simulink model "laby2"  (R2016a)
settings: Solver=ode23  StartTime=0.0  StopTime=10.0  RelTol=1e-5
libraries: simulink x2
settings Model: Creator=wojta  LastModifiedBy=wojta

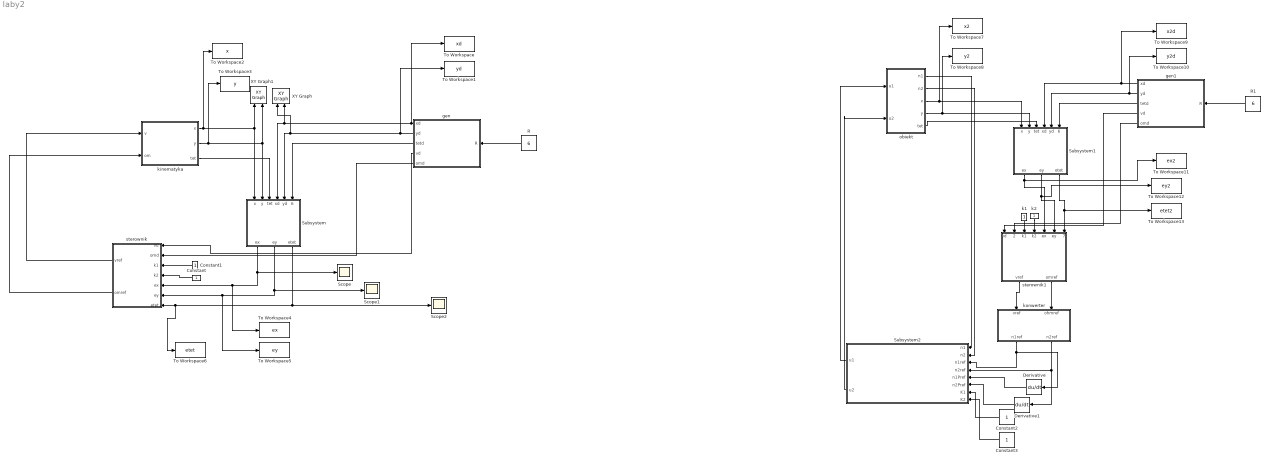
== system laby2 ==
  Constant{,1..3} (4 alike) : Constant
  Derivative : Derivative
  Derivative1 : Derivative
  R : Constant  Value=6
  R1 : Constant  Value=6
  Scope : Scope
  Scope1 : Scope
  Scope2 : Scope
  Subsystem : Subsystem
  Subsystem1 : Subsystem
  Subsystem2 : Subsystem
  To Workspace : ToWorkspace  VariableName=xd  SampleTime=-1
  To Workspace1 : ToWorkspace  VariableName=yd  SampleTime=-1
  To Workspace10 : ToWorkspace  VariableName=y2d  SampleTime=-1
  To Workspace11 : ToWorkspace  VariableName=ex2  SampleTime=-1
  To Workspace12 : ToWorkspace  VariableName=ey2  SampleTime=-1
  To Workspace13 : ToWorkspace  VariableName=etet2  SampleTime=-1
  To Workspace2 : ToWorkspace  VariableName=x  SampleTime=-1
  To Workspace3 : ToWorkspace  VariableName=y  SampleTime=-1
  To Workspace4 : ToWorkspace  VariableName=ex  SampleTime=-1
  To Workspace5 : ToWorkspace  VariableName=ey  SampleTime=-1
  To Workspace6 : ToWorkspace  VariableName=etet  SampleTime=-1
  To Workspace7 : ToWorkspace  VariableName=x2  SampleTime=-1
  To Workspace8 : ToWorkspace  VariableName=y2  SampleTime=-1
  To Workspace9 : ToWorkspace  VariableName=x2d  SampleTime=-1
  XY Graph : simulink/Sinks/XY Graph  xmin=-6  xmax=6  ymin=-6  ymax=6  st=-1
  XY Graph1 : simulink/Sinks/XY Graph  xmin=-6  xmax=6  ymin=-6  ymax=6  st=-1
  gen : Subsystem
  gen1 : Subsystem
  k1 : Constant
  k2 : Constant
  kinematyka : Subsystem
  konwerter : Subsystem
  obiekt : Subsystem
  sterownik : Subsystem
  sterownik1 : Subsystem
  wires:
  R/1 -> gen/1(R)
  sterownik/1(vref) -> kinematyka/1(v)
  sterownik/2(omref) -> kinematyka/2(om)
  kinematyka/1(x) -> To Workspace2/1, XY Graph1/1, Subsystem/1(x)
  kinematyka/2(y) -> To Workspace3/1, XY Graph1/2, Subsystem/2(y)
  kinematyka/3(tet) -> Subsystem/3(tet)
  gen/1(xd) -> To Workspace/1, XY Graph/2, Subsystem/4(xd)
  gen/2(yd) -> To Workspace1/1, XY Graph/1, Subsystem/5(yd)
  gen/3(tetd) -> Subsystem/6(tetd)
  Subsystem/1(ex) -> To Workspace4/1, sterownik/5(ex), Scope/1
  Subsystem/2(ey) -> To Workspace5/1, sterownik/6(ey), Scope1/1
  Subsystem/3(etet) -> Scope2/1, To Workspace6/1, sterownik/7(etet)
  gen/4(vd) -> sterownik/1(vd)
  gen/5(omd) -> sterownik/2(omd)
  Constant1/1 -> sterownik/3(k1)
  Constant/1 -> sterownik/4(k2)
  R1/1 -> gen1/1(R)
  k2/1 -> sterownik1/4(k2)
  k1/1 -> sterownik1/3(k1)
  Subsystem1/3(etet) -> sterownik1/7(etet), To Workspace13/1
  Subsystem1/2(ey) -> To Workspace12/1, sterownik1/6(ey)
  Subsystem1/1(ex) -> To Workspace11/1, sterownik1/5(ex)
  gen1/4(vd) -> sterownik1/1(vd)
  gen1/5(omd) -> sterownik1/2(omd)
  gen1/2(yd) -> To Workspace10/1, Subsystem1/5(yd)
  gen1/3(tetd) -> Subsystem1/6(tetd)
  obiekt/3(x) -> To Workspace7/1, Subsystem1/1(x)
  obiekt/4(y) -> To Workspace8/1, Subsystem1/2(y)
  obiekt/5(tet) -> Subsystem1/3(tet)
  sterownik1/1(vref) -> konwerter/1(vref)
  sterownik1/2(omref) -> konwerter/2(ohmref)
  konwerter/1(n1ref) -> Derivative/1, Subsystem2/3(n1ref)
  konwerter/2(n2ref) -> Derivative1/1, Subsystem2/4(n2ref)
  Derivative/1 -> Subsystem2/5(n1Pref)
  Derivative1/1 -> Subsystem2/6(n2Pref)
  Subsystem2/1(u1) -> obiekt/1(u1)
  Subsystem2/2(u2) -> obiekt/2(u2)
  obiekt/2(n2) -> Subsystem2/2(n2)
  obiekt/1(n1) -> Subsystem2/1(n1)
  Constant2/1 -> Subsystem2/7(K1)
  Constant3/1 -> Subsystem2/8(K2)
  gen1/1(xd) -> To Workspace9/1, Subsystem1/4(xd)

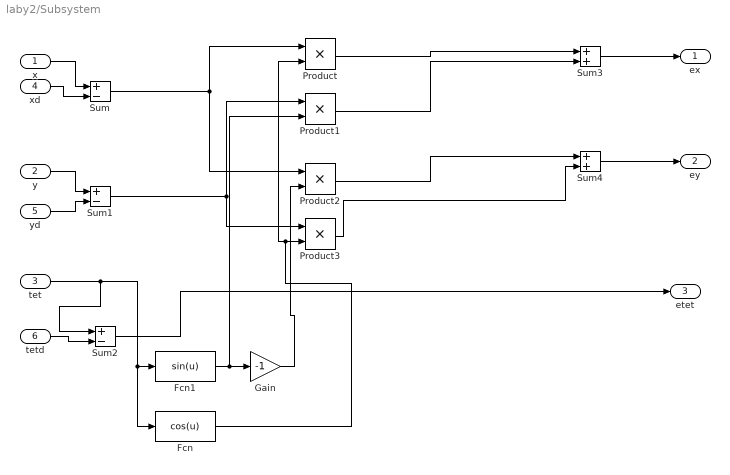
== system laby2/Subsystem ==
  x : Inport
  y : Inport  Port=2
  tet : Inport  Port=3
  xd : Inport  Port=4
  yd : Inport  Port=5
  tetd : Inport  Port=6
  Fcn : Fcn  Expr=cos(u)
  Fcn1 : Fcn  Expr=sin(u)
  Gain : Gain  Gain=-1
  Product{,1..3} (4 alike) : Product
  Sum : Sum  Inputs=+-
  Sum1 : Sum  Inputs=+-
  Sum2 : Sum  Inputs=+-
  Sum3 : Sum
  Sum4 : Sum
  ex : Outport
  ey : Outport  Port=2
  etet : Outport  Port=3
  wires:
  xd/1 -> Sum/2
  yd/1 -> Sum1/2
  Product3/1 -> Sum4/2
  tetd/1 -> Sum2/2
  Fcn1/1 -> Product1/2, Gain/1
  Product1/1 -> Sum3/2
  tet/1 -> Fcn/1, Fcn1/1, Sum2/1
  Gain/1 -> Product2/2
  Product2/1 -> Sum4/1
  Sum2/1 -> etet/1
  y/1 -> Sum1/1
  Product/1 -> Sum3/1
  Sum1/1 -> Product3/1, Product1/1
  Sum4/1 -> ey/1
  x/1 -> Sum/1
  Fcn/1 -> Product/2, Product3/2
  Sum3/1 -> ex/1
  Sum/1 -> Product/1, Product2/1

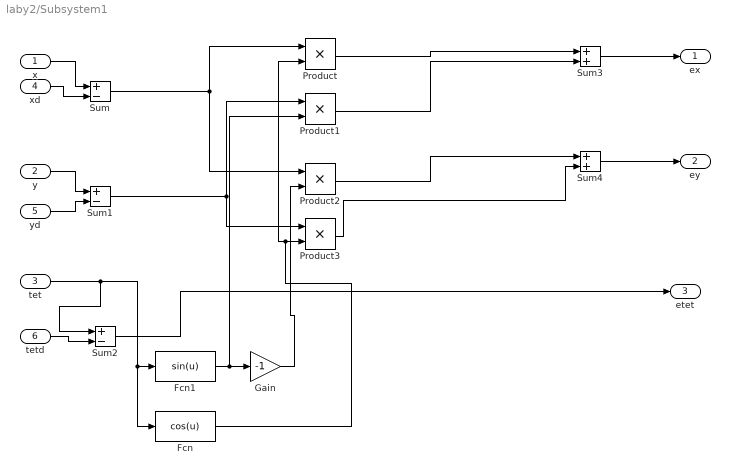
== system laby2/Subsystem1 ==
  x : Inport
  y : Inport  Port=2
  tet : Inport  Port=3
  xd : Inport  Port=4
  yd : Inport  Port=5
  tetd : Inport  Port=6
  Fcn : Fcn  Expr=cos(u)
  Fcn1 : Fcn  Expr=sin(u)
  Gain : Gain  Gain=-1
  Product{,1..3} (4 alike) : Product
  Sum : Sum  Inputs=+-
  Sum1 : Sum  Inputs=+-
  Sum2 : Sum  Inputs=+-
  Sum3 : Sum
  Sum4 : Sum
  ex : Outport
  ey : Outport  Port=2
  etet : Outport  Port=3
  wires:
  xd/1 -> Sum/2
  yd/1 -> Sum1/2
  Product3/1 -> Sum4/2
  tetd/1 -> Sum2/2
  Fcn1/1 -> Product1/2, Gain/1
  Product1/1 -> Sum3/2
  tet/1 -> Fcn/1, Fcn1/1, Sum2/1
  Gain/1 -> Product2/2
  Product2/1 -> Sum4/1
  Sum2/1 -> etet/1
  y/1 -> Sum1/1
  Product/1 -> Sum3/1
  Sum1/1 -> Product3/1, Product1/1
  Sum4/1 -> ey/1
  x/1 -> Sum/1
  Fcn/1 -> Product/2, Product3/2
  Sum3/1 -> ex/1
  Sum/1 -> Product/1, Product2/1

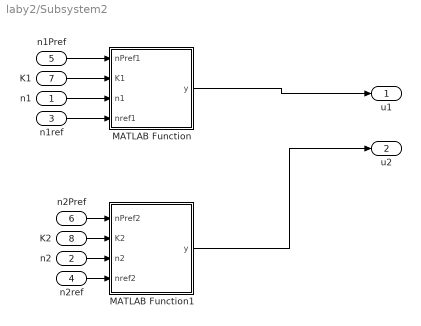
== system laby2/Subsystem2 ==
  n1 : Inport
  n2 : Inport  Port=2
  n1ref : Inport  Port=3
  n2ref : Inport  Port=4
  n1Pref : Inport  Port=5
  n2Pref : Inport  Port=6
  K1 : Inport  Port=7
  K2 : Inport  Port=8
  MATLAB Function : MATLAB Function  TreatAsAtomicUnit=on
  MATLAB Function1 : MATLAB Function  TreatAsAtomicUnit=on
  u1 : Outport
  u2 : Outport  Port=2
  wires:
  MATLAB Function/1(y) -> u1/1
  MATLAB Function1/1(y) -> u2/1
  n1Pref/1 -> MATLAB Function/1(nPref1)
  K1/1 -> MATLAB Function/2(K1)
  n1/1 -> MATLAB Function/3(n1)
  n1ref/1 -> MATLAB Function/4(nref1)
  n2Pref/1 -> MATLAB Function1/1(nPref2)
  K2/1 -> MATLAB Function1/2(K2)
  n2/1 -> MATLAB Function1/3(n2)
  n2ref/1 -> MATLAB Function1/4(nref2)

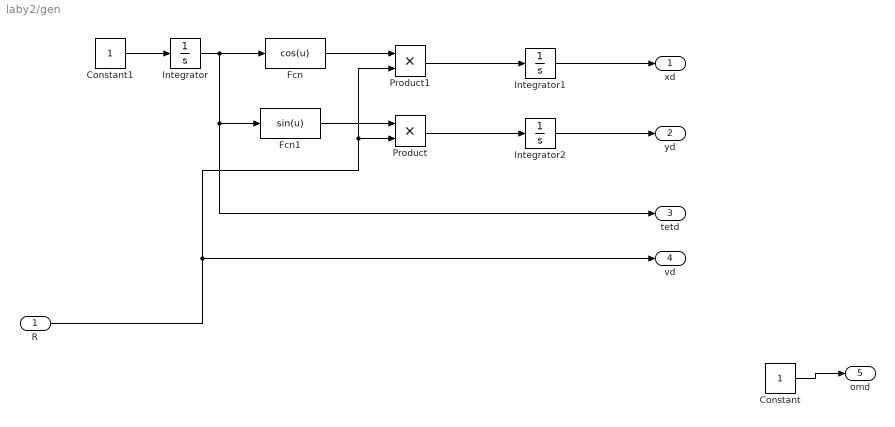
== system laby2/gen ==
  R : Inport
  Constant : Constant
  Constant1 : Constant
  Fcn : Fcn  Expr=cos(u)
  Fcn1 : Fcn  Expr=sin(u)
  Integrator : Integrator
  Integrator1 : Integrator
  Integrator2 : Integrator  InitialCondition=-6
  Product : Product
  Product1 : Product
  xd : Outport
  yd : Outport  Port=2
  tetd : Outport  Port=3
  vd : Outport  Port=4
  omd : Outport  Port=5
  wires:
  Constant/1 -> omd/1
  R/1 -> Product1/2, Product/2, vd/1
  Constant1/1 -> Integrator/1
  Integrator/1 -> Fcn1/1, tetd/1, Fcn/1
  Fcn1/1 -> Product/1
  Fcn/1 -> Product1/1
  Product/1 -> Integrator2/1
  Product1/1 -> Integrator1/1
  Integrator1/1 -> xd/1
  Integrator2/1 -> yd/1

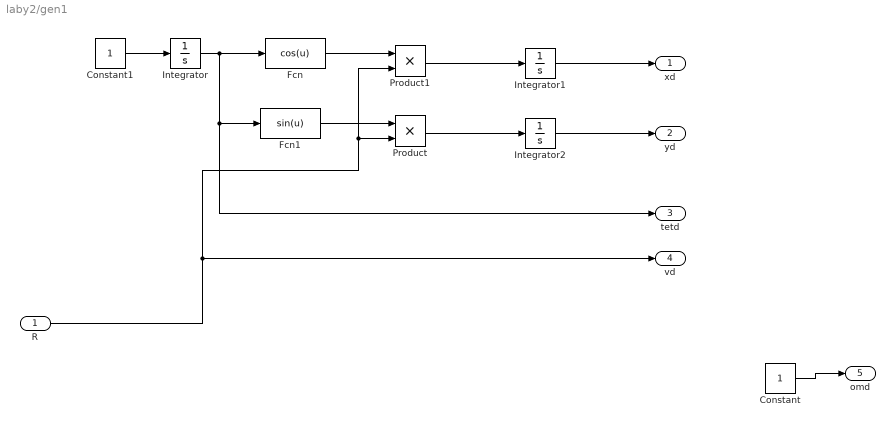
== system laby2/gen1 ==
  R : Inport
  Constant : Constant
  Constant1 : Constant
  Fcn : Fcn  Expr=cos(u)
  Fcn1 : Fcn  Expr=sin(u)
  Integrator : Integrator
  Integrator1 : Integrator
  Integrator2 : Integrator  InitialCondition=-6
  Product : Product
  Product1 : Product
  xd : Outport
  yd : Outport  Port=2
  tetd : Outport  Port=3
  vd : Outport  Port=4
  omd : Outport  Port=5
  wires:
  Constant/1 -> omd/1
  R/1 -> Product1/2, Product/2, vd/1
  Constant1/1 -> Integrator/1
  Integrator/1 -> Fcn1/1, tetd/1, Fcn/1
  Fcn1/1 -> Product/1
  Fcn/1 -> Product1/1
  Product/1 -> Integrator2/1
  Product1/1 -> Integrator1/1
  Integrator1/1 -> xd/1
  Integrator2/1 -> yd/1

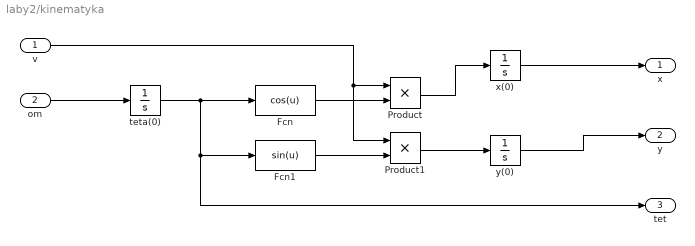
== system laby2/kinematyka ==
  v : Inport
  om : Inport  Port=2
  Fcn : Fcn  Expr=cos(u)
  Fcn1 : Fcn  Expr=sin(u)
  Product : Product
  Product1 : Product
  teta(0) : Integrator
  x(0) : Integrator  InitialCondition=1
  y(0) : Integrator  InitialCondition=1
  x : Outport
  y : Outport  Port=2
  tet : Outport  Port=3
  wires:
  Fcn1/1 -> Product1/2
  teta(0)/1 -> tet/1, Fcn1/1, Fcn/1
  x(0)/1 -> x/1
  om/1 -> teta(0)/1
  Product1/1 -> y(0)/1
  y(0)/1 -> y/1
  Fcn/1 -> Product/2
  Product/1 -> x(0)/1
  v/1 -> Product1/1, Product/1

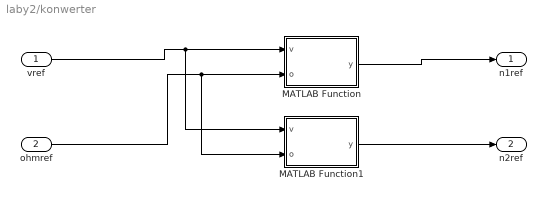
== system laby2/konwerter ==
  vref : Inport
  ohmref : Inport  Port=2
  MATLAB Function : MATLAB Function  TreatAsAtomicUnit=on
  MATLAB Function1 : MATLAB Function  TreatAsAtomicUnit=on
  n1ref : Outport
  n2ref : Outport  Port=2
  wires:
  MATLAB Function/1(y) -> n1ref/1
  vref/1 -> MATLAB Function1/1(v), MATLAB Function/1(v)
  ohmref/1 -> MATLAB Function1/2(o), MATLAB Function/2(o)
  MATLAB Function1/1(y) -> n2ref/1

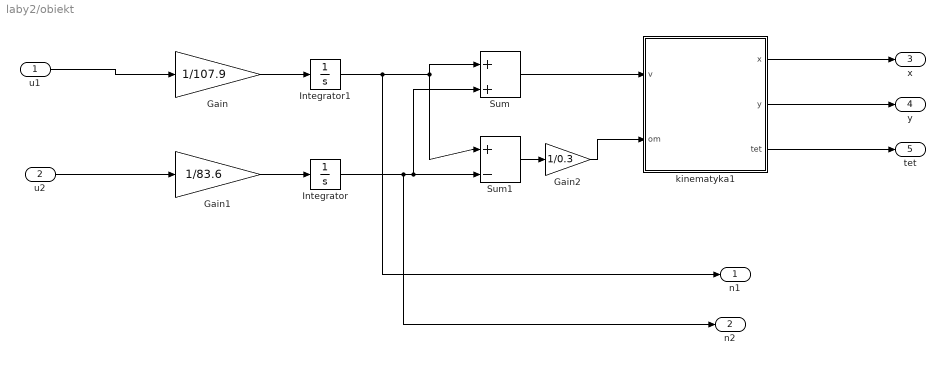
== system laby2/obiekt ==
  u1 : Inport
  u2 : Inport  Port=2
  Gain : Gain  Gain=1/107.9
  Gain1 : Gain  Gain=1/83.6
  Gain2 : Gain  Gain=1/0.3
  Integrator : Integrator
  Integrator1 : Integrator
  Sum : Sum  Inputs=|++
  Sum1 : Sum  Inputs=|+-
  kinematyka1 : Subsystem
  n1 : Outport
  n2 : Outport  Port=2
  x : Outport  Port=3
  y : Outport  Port=4
  tet : Outport  Port=5
  wires:
  Integrator1/1 -> n1/1, Sum1/1, Sum/1
  Sum1/1 -> Gain2/1
  Gain/1 -> Integrator1/1
  kinematyka1/3(tet) -> tet/1
  kinematyka1/2(y) -> y/1
  u1/1 -> Gain/1
  u2/1 -> Gain1/1
  Integrator/1 -> n2/1, Sum1/2, Sum/2
  Gain1/1 -> Integrator/1
  Sum/1 -> kinematyka1/1(v)
  kinematyka1/1(x) -> x/1
  Gain2/1 -> kinematyka1/2(om)

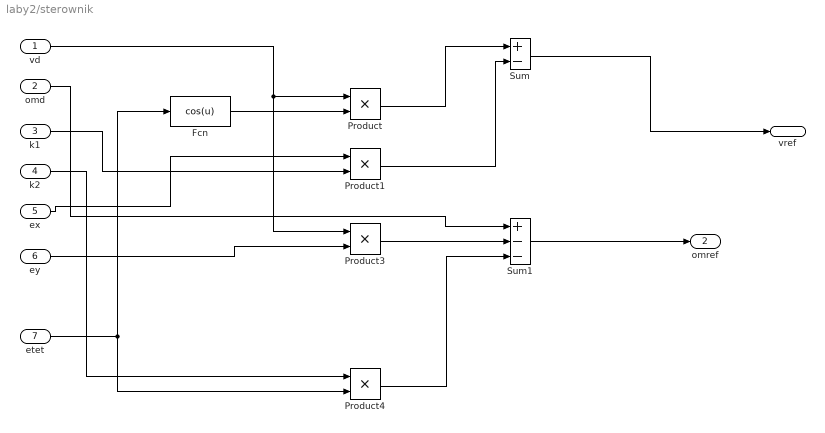
== system laby2/sterownik ==
  vd : Inport
  omd : Inport  Port=2
  k1 : Inport  Port=3
  k2 : Inport  Port=4
  ex : Inport  Port=5
  ey : Inport  Port=6
  etet : Inport  Port=7
  Fcn : Fcn  Expr=cos(u)
  Product{,1,3..4} (4 alike) : Product
  Sum : Sum  Inputs=+-
  Sum1 : Sum  Inputs=+--
  vref : Outport
  omref : Outport  Port=2
  wires:
  ex/1 -> Product1/1
  Product4/1 -> Sum1/3
  Sum1/1 -> omref/1
  k1/1 -> Product1/2
  ey/1 -> Product3/2
  etet/1 -> Fcn/1, Product4/2
  omd/1 -> Sum1/1
  Product3/1 -> Sum1/2
  Fcn/1 -> Product/2
  vd/1 -> Product3/1, Product/1
  k2/1 -> Product4/1
  Sum/1 -> vref/1
  Product1/1 -> Sum/2
  Product/1 -> Sum/1

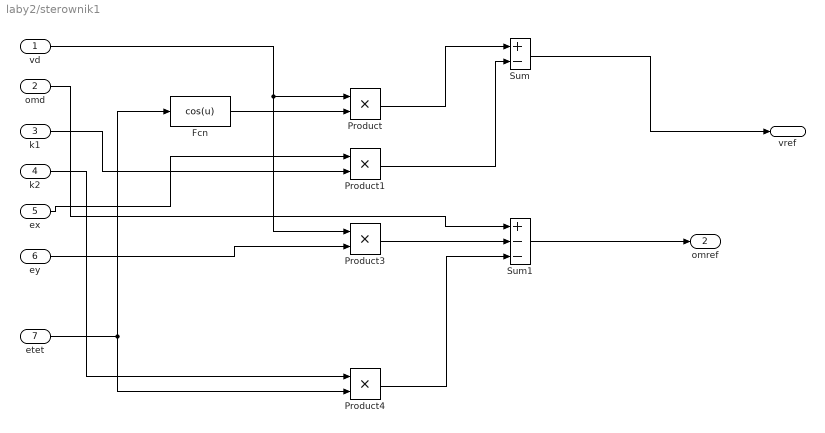
== system laby2/sterownik1 ==
  vd : Inport
  omd : Inport  Port=2
  k1 : Inport  Port=3
  k2 : Inport  Port=4
  ex : Inport  Port=5
  ey : Inport  Port=6
  etet : Inport  Port=7
  Fcn : Fcn  Expr=cos(u)
  Product{,1,3..4} (4 alike) : Product
  Sum : Sum  Inputs=+-
  Sum1 : Sum  Inputs=+--
  vref : Outport
  omref : Outport  Port=2
  wires:
  ex/1 -> Product1/1
  Product4/1 -> Sum1/3
  Sum1/1 -> omref/1
  k1/1 -> Product1/2
  ey/1 -> Product3/2
  etet/1 -> Fcn/1, Product4/2
  omd/1 -> Sum1/1
  Product3/1 -> Sum1/2
  Fcn/1 -> Product/2
  vd/1 -> Product3/1, Product/1
  k2/1 -> Product4/1
  Sum/1 -> vref/1
  Product1/1 -> Sum/2
  Product/1 -> Sum/1

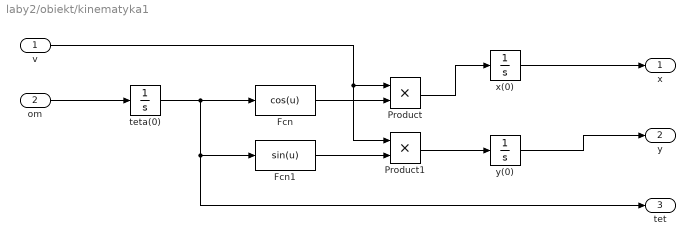
== system laby2/obiekt/kinematyka1 ==
  v : Inport
  om : Inport  Port=2
  Fcn : Fcn  Expr=cos(u)
  Fcn1 : Fcn  Expr=sin(u)
  Product : Product
  Product1 : Product
  teta(0) : Integrator
  x(0) : Integrator  InitialCondition=1
  y(0) : Integrator  InitialCondition=1
  x : Outport
  y : Outport  Port=2
  tet : Outport  Port=3
  wires:
  Fcn1/1 -> Product1/2
  teta(0)/1 -> tet/1, Fcn1/1, Fcn/1
  x(0)/1 -> x/1
  om/1 -> teta(0)/1
  Product1/1 -> y(0)/1
  y(0)/1 -> y/1
  Fcn/1 -> Product/2
  Product/1 -> x(0)/1
  v/1 -> Product1/1, Product/1

== matlab function laby2/konwerter/MATLAB Function1 ==
  data: v input; y output; o input
function y = fcn(v, o)
%#codegen

y = 0.5*(v-0.3*o);

== matlab function laby2/konwerter/MATLAB Function ==
  data: v input; y output; o input
function y = fcn(v, o)
%#codegen

y = 0.5*(v+0.3*o);

== matlab function laby2/Subsystem2/MATLAB Function ==
  data: nPref1 input; y output; K1 input; n1 input; nref1 input
function y = fcn(nPref1, K1, n1, nref1)
%#codegen

y = 107.9*nPref1-K1*(n1-nref1);

== matlab function laby2/Subsystem2/MATLAB Function1 ==
  data: nPref2 input; y output; K2 input; n2 input; nref2 input
function y = fcn(nPref2, K2, n2, nref2)
%#codegen

y = 83.6*nPref2-K2*(n2-nref2);
